simulink model "CascadePID"  (R2016b)
settings: Solver=ode5  StartTime=0.0  StopTime=10  FixedStep=1e-4  RelTol=1e-3
settings Model: Creator=Admin  LastModifiedBy=Admin

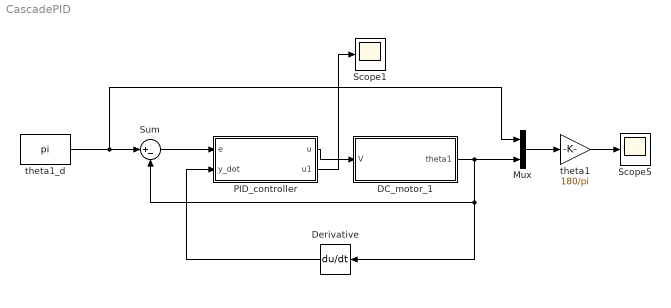
== system CascadePID ==
  DC_motor_1 : Subsystem  mask{Ki=0.043, Kb=0.04297, L=0.0001, R=1.025, Jeff=0.000056+(1e-4)*5, Beff=0.00008092, N=100}
  Derivative : Derivative
  Mux : Mux  Inputs=2
  PID_controller : Subsystem  mask{Kpp=5, Kp=10, Ki=50}
  Scope1 : Scope
  Scope5 : Scope
  Sum : Sum  Inputs=|+-
  theta1 : Gain  Gain=180/pi
  theta1_d : Constant  Value=pi
  wires:
  Sum/1 -> PID_controller/1(e)
  PID_controller/1(u) -> DC_motor_1/1(V)
  theta1_d/1 -> Mux/1, Sum/1
  DC_motor_1/1(theta1) -> Mux/2, Derivative/1, Sum/2
  Derivative/1 -> PID_controller/2(y_dot)
  Mux/1 -> theta1/1
  theta1/1 -> Scope5/1
  PID_controller/2(u1) -> Scope1/1

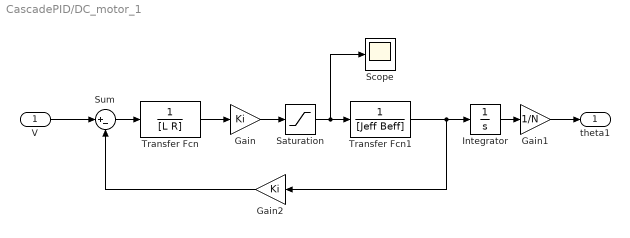
== system CascadePID/DC_motor_1 ==
  V : Inport
  Gain : Gain  Gain=Ki
  Gain1 : Gain  Gain=1/N
  Gain2 : Gain  Gain=Ki
  Integrator : Integrator
  Saturation : Saturate  UpperLimit=4  LowerLimit=-4
  Scope : Scope
  Sum : Sum  Inputs=|+-
  Transfer Fcn : TransferFcn  Denominator=[L R]
  Transfer Fcn1 : TransferFcn  Denominator=[Jeff Beff]
  theta1 : Outport
  wires:
  Sum/1 -> Transfer Fcn/1
  Transfer Fcn/1 -> Gain/1
  Gain/1 -> Saturation/1
  Transfer Fcn1/1 -> Integrator/1, Gain2/1
  Integrator/1 -> Gain1/1
  Gain1/1 -> theta1/1
  Gain2/1 -> Sum/2
  V/1 -> Sum/1
  Saturation/1 -> Scope/1, Transfer Fcn1/1

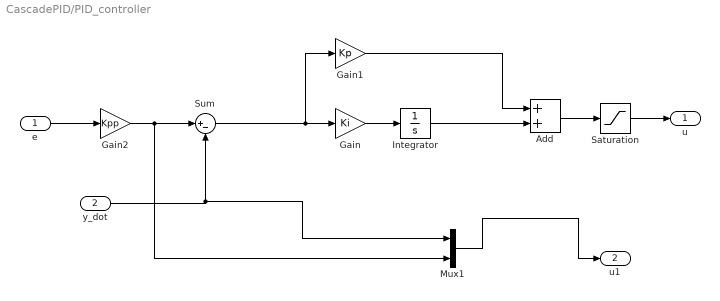
== system CascadePID/PID_controller ==
  e : Inport
  y_dot : Inport  Port=2
  Add : Sum
  Gain : Gain  Gain=Ki
  Gain1 : Gain  Gain=Kp
  Gain2 : Gain  Gain=Kpp
  Integrator : Integrator
  Mux1 : Mux  Inputs=2
  Saturation : Saturate  UpperLimit=48  LowerLimit=-48
  Sum : Sum  Inputs=|+-
  u : Outport
  u1 : Outport  Port=2
  wires:
  e/1 -> Gain2/1
  Gain/1 -> Integrator/1
  Gain1/1 -> Add/1
  Integrator/1 -> Add/2
  Add/1 -> Saturation/1
  Saturation/1 -> u/1
  Sum/1 -> Gain1/1, Gain/1
  Gain2/1 -> Mux1/2, Sum/1
  Mux1/1 -> u1/1
  y_dot/1 -> Mux1/1, Sum/2
